simulink model "MPPT(P_O)v1"  (R2019b)
settings: Solver=VariableStepAuto  StartTime=0.0  StopTime=1.5  RelTol=1e-3
libraries: powerlib x7, re_lib x1, powerlib_meascontrol x1, simulink x1
settings Model: Creator=Dell  LastModifiedBy=Dell

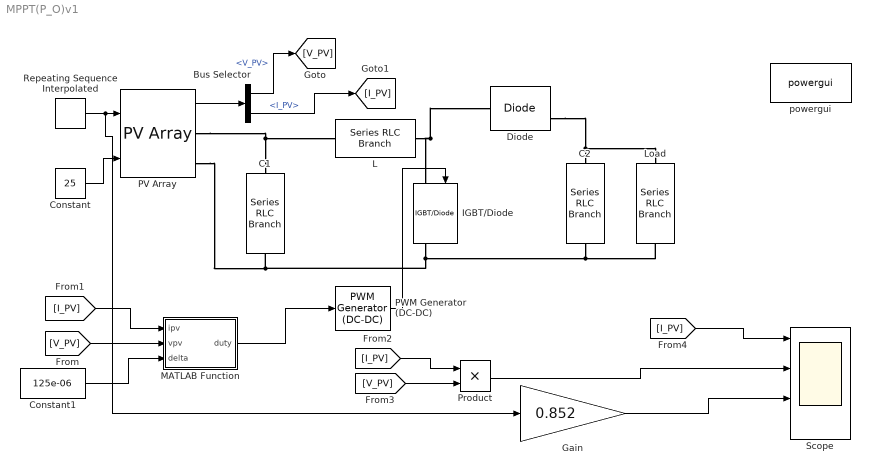
== system MPPT(P_O)v1 ==
  Bus Selector : BusSelector  OutputSignals=V_PV,I_PV
  C1 : powerlib/Elements/Series RLC Branch  LConnTagsString=__new0  RConnTagsString=__new0  BranchType=RC  Resistance=1e-4  Inductance=1e-3  SetiL0=off  InitialCurrent=0  Capacitance=100e-6  Setx0=off  InitialVoltage=0  Measurements=None
      settings: SourceProductName=Simscape Electrical
  C2 : powerlib/Elements/Series RLC Branch  LConnTagsString=__new0  RConnTagsString=__new0  BranchType=RC  Resistance=1e-4  Inductance=1e-3  SetiL0=off  InitialCurrent=0  Capacitance=100e-6  Setx0=off  InitialVoltage=0  Measurements=None
      settings: SourceProductName=Simscape Electrical
  Constant : Constant  Value=25
  Constant1 : Constant  Value=125e-06
  Diode : powerlib/Power Electronics/Diode  Ron=0.001  Lon=0  Vf=0.8  IC=0  UseSnubber=0  Rs=500  Cs=250e-9  Measurements=on
      settings: SourceProductName=Simscape Electrical
  Gain : Gain  Gain=0.852
  IGBT/Diode : powerlib/Power Electronics/IGBT//Diode  Ron=1e-3  Rs=1e5  Cs=inf  Measurements=on
      settings: SourceProductName=Simscape Electrical
  L : powerlib/Elements/Series RLC Branch  LConnTagsString=__new0  RConnTagsString=__new0  BranchType=RL  Resistance=0.1  Inductance=2e-3  SetiL0=off  InitialCurrent=0  Capacitance=1e-6  Setx0=off  InitialVoltage=0  Measurements=None
      settings: SourceProductName=Simscape Electrical
  Load : powerlib/Elements/Series RLC Branch  LConnTagsString=__new0  RConnTagsString=__new0  BranchType=R  Resistance=400  Inductance=1e-3  SetiL0=off  InitialCurrent=0  Capacitance=1e-6  Setx0=off  InitialVoltage=0  Measurements=None
      settings: SourceProductName=Simscape Electrical
  MATLAB Function : MATLAB Function  TreatAsAtomicUnit=on
  PV Array : re_lib/Solar/PV Array  Npar=2  Nser=2  PlotType=array @ 1000 W/m2 & specified temperatures  S_vec="[ 1000  500  100 ]"  Temp_C_vec="[ 45 25  ]"  ModuleName=1Soltech 1STH-215-P  PlotWhenSelected=off  Pm=213.15  Ncell=60  Voc=36.3  Isc=7.84  Vm=29  Im=7.35  beta_Voc_pc=-0.36099  alpha_Isc_pc=0.102  beta_Voc=-0.13104  alpha_Isc=0.007997  IL=7.8649  I0=2.9259e-10  nI=0.98117  Rsh=313.3991  Rs=0.39383  BAL=off  Tc=1e-6  Tfilter=5e-5
      settings: SourceProductName=Simscape Electrical
  PWM Generator (DC-DC) : powerlib_meascontrol/Pulse & Signal Generators/PWM Generator (DC-DC)  Fsw=5000  Ts=0
      settings: SourceProductName=Simscape Electrical
  Product : Product
  Repeating Sequence Interpolated : simulink/Sources/Repeating Sequence Interpolated  OutValues=[0 300 500 1000 1000 500 500 300 300 0].'  TimeValues="[0 0.25 0.2501 0.5 0.51 0.75 1.01 1.25 1.2501 1.5  ].'"  LookUpMeth=Interpolation-Use End Values  tsamp=5e-06  OutMin=[]  OutMax=[]  OutDataTypeStr=double  OutputDataTypeScalingMode=double  OutDataType=fixdt(0,8)  OutScaling=2^-10
  Scope : Scope  NumInputPorts=4
  powergui : powerlib/powergui  Priority=1  SimulationMode=Discrete  SampleTime=5e-6  frequency=60  Iterations=50  frequencyindice=0  Pbase=100e6  ErrMax=1e-4  UnitsV=kV  UnitsW=MW  buscounter=0  FunctionMessages=off  echomessages=off  EnableUseOfTLC=off  CurrentSourceSwitches=off  DisableSnubberDevices=off  DisableRonSwitches=off  DisableVfSwitches=off  DisplayEquations=off  AutomaticDiscreteSolvers=off  SolverType=Tustin/Backward Euler (TBE)  Interpol=off  ExternalGateDelay=off  methode=off  Ts=100  x0status=blocks  SPID=on  SwTol=0  HookPort=off  NonlinearTolerance=1e-4  nMaxIteration=100  ContinueOnMaxIteration=off  RestoreLinks=warning  ResistiveCurrentMeasurement=off  Frange=[0:2:500]  Ylog=off  Xlog=on  ShowGrid=off  save=off  variable=ZData  structure=0  ZoomFFT=off  StartTime=0.0  cycles=1  DisplayStyle=1  fundamental=60  FreqAxis=off  MaxFrequency=1000  frequencyindicesteady=1  RmsSteady=1  display=off
      settings: SourceProductName=Simscape Electrical
  wires:
  PV Array/1 -> Bus Selector/1
  Repeating Sequence Interpolated/1 -> Gain/1, PV Array/1
  Constant/1 -> PV Array/2
  PWM Generator (DC-DC)/1 -> IGBT/Diode/1
  Bus Selector/1 -> [V_PV]  "<V_PV>"
  Bus Selector/2 -> [I_PV]  "<I_PV>"
  MATLAB Function/1(duty) -> PWM Generator (DC-DC)/1
  Constant1/1 -> MATLAB Function/3(delta)
  [I_PV] -> Product/1
  [V_PV] -> Product/2
  [I_PV] -> Scope/1
  [I_PV] -> MATLAB Function/1(ipv)
  [V_PV] -> MATLAB Function/2(vpv)
  Product/1 -> Scope/2
  Gain/1 -> Scope/3
  connections:
  PV Array/RConn1 -- L/LConn1 -- C1/LConn1
  L/RConn1 -- IGBT/Diode/LConn1 -- Diode/LConn1
  IGBT/Diode/RConn1 -- C2/RConn1 -- Load/RConn1 -- PV Array/RConn2 -- C1/RConn1
  Diode/RConn1 -- Load/LConn1 -- C2/LConn1

== matlab function MPPT(P_O)v1/MATLAB Function ==
  data: ipv input; duty output; vpv input; delta input
function duty = MPPT(ipv,vpv,delta)
duty_int=0.1;
duty_max=0.9;
duty_min=0;

persistent Vold Pold Dold;
if isempty(Vold)
    Vold=0;
    Pold=0;
    Dold=duty_int;
end


Piv=ipv*vpv;
delP=Piv-Pold;
delV=vpv-Vold;
if(delP~=0)
    
    if(delP>0)
        if(delV>0)
            duty=Dold-delta;
        else
            duty=Dold+delta;
        end

    else
        if(delV>0)
            duty=Dold+delta;
        else
            duty=Dold-delta;
        end
    end
    
else
    duty=Dold;
end

if(duty>duty_max)
    duty=duty_max;
elseif(duty<duty_min)
    duty=duty_min;
end
   
    
    
    Vold=vpv;
    Pold=Piv;
    Dold=duty;
